simulink model "base_01"  (Simulink 8.6)
settings: Solver=VariableStepAuto  StartTime=0.0  StopTime=3  MaxStep=0.000001  RelTol=1e-3
undefined symbols (not defined in the file or in its folder): delay
libraries: commsynccomp2 x1, simulink x1
settings Model: Creator=my88899  LastModifiedBy=my88899
settings SolverCC: InitialStep=0.000001
settings DataIOCC: SaveFormat=Dataset  SignalLoggingSaveFormat=Dataset
settings OptimizationCC: ExpressionDepthLimit=128
settings DebuggingCC: UnderspecifiedInitializationDetection=Simplified  MergeDetectMultiDrivingBlocksExec=error  SolverPrmCheckMsg=none  FcnCallInpInsideContextMsg=EnableAllAsError  StateNameClashWarn=none
settings HardwareCC: ProdBitPerPointer=64  ProdLargestAtomicFloat=Float  ProdIntDivRoundTo=Zero  ProdEndianess=LittleEndian  ProdWordSize=64  ProdHWDeviceType=Intel->x86-64 (Windows64)
settings GRTTargetCC: GeneratePreprocessorConditionals=Use local settings  CombineOutputUpdateFcns=on  GRTInterface=off
settings ConfigComp: CovModelRefEnable=off
settings ConfigurationSet: Description=SimMechanics 2G

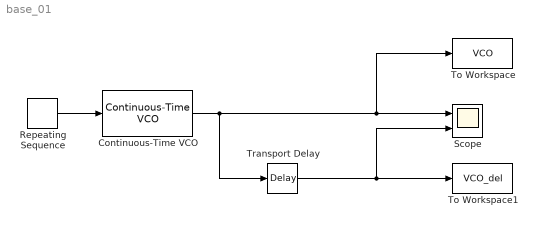
== system base_01 ==
  Continuous-Time VCO : commsynccomp2/Continuous-Time VCO  Ac=5  Fc=1000  Kc=1000  Ph=0
  Repeating Sequence : simulink/Sources/Repeating Sequence  rep_seq_t=[0 1]  rep_seq_y=[0 10]
  Scope : Scope  NumInputPorts=2
  To Workspace : ToWorkspace  VariableName=VCO  SaveFormat=Timeseries  SampleTime=-1
  To Workspace1 : ToWorkspace  VariableName=VCO_del  SaveFormat=Timeseries  SampleTime=-1
  Transport Delay : TransportDelay  DelayTime=delay  BufferSize=3000000
  wires:
  Repeating Sequence/1 -> Continuous-Time VCO/1
  Continuous-Time VCO/1 -> Transport Delay/1, To Workspace/1, Scope/1
  Transport Delay/1 -> To Workspace1/1, Scope/2
